simulink model "dc_motor"  (R2021a)
settings: Solver=FixedStepAuto  StartTime=0.0  StopTime=10  FixedStep=0.1  RelTol=1e-3
model workspace (MAT data in the model file):
  B = Simulink.Parameter
  B.Value = 0.2
  B.DataType = 'auto'
  B.Min = 0
  B.Dimensions = [1 1]
  J = Simulink.Parameter
  J.Value = 0.02
  J.DataType = 'auto'
  J.Min = 0
  J.Dimensions = [1 1]
  K = Simulink.Parameter
  K.Value = 0.1
  K.DataType = 'auto'
  K.Min = 0
  K.Dimensions = [1 1]
  L = Simulink.Parameter
  L.Value = 0.5
  L.DataType = 'auto'
  L.Min = 0
  L.Dimensions = [1 1]
  R = Simulink.Parameter
  R.Value = 2
  R.DataType = 'auto'
  R.Min = 0
  R.Dimensions = [1 1]
settings Model: OrderedModelArguments=off  Creator=WALEED ELBADRY  LastModifiedBy=WALEED ELBADRY

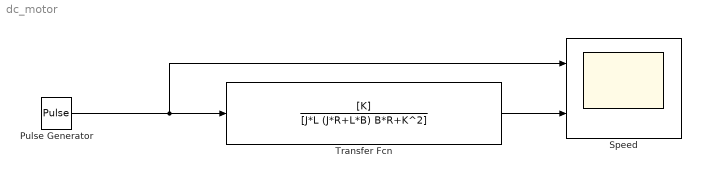
== system dc_motor ==
  Pulse Generator : DiscretePulseGenerator  Amplitude=0.2  Period=20  PulseWidth=10  PhaseDelay=10  SampleTime=0.1
  Speed : Scope  NumInputPorts=2
  Transfer Fcn : TransferFcn  Numerator=[K]  Denominator=[J*L (J*R+L*B) B*R+K^2]  ContinuousStateAttributes='speed'
  wires:
  Pulse Generator/1 -> Speed/1, Transfer Fcn/1
  Transfer Fcn/1 -> Speed/2
